simulink model "singleinvertedpendulumsim"  (R2018a)
settings: Solver=FixedStepDiscrete  StartTime=0.0  StopTime=Tsim  FixedStep=Ts  RelTol=1e-3
values from neighbouring files (symbols this model uses):
  K2 = -K2    [singleinvertedpendulum.m]
  R = 0.021    [singleinvertedpendulum.m]
  Ts = 0.001    [singleinvertedpendulum.m]
  x0 = [0;0.1;0;0]    [singleinvertedpendulum.m]
undefined symbols (not defined in the file or in its folder): Ad, Bd, Cd, Dd, Discrete, Ed, Fd, Gd, Hd, Time
libraries: ctrlSharedLib x1, simulink x1
settings Model: Creator=srivats  LastModifiedBy=srivats

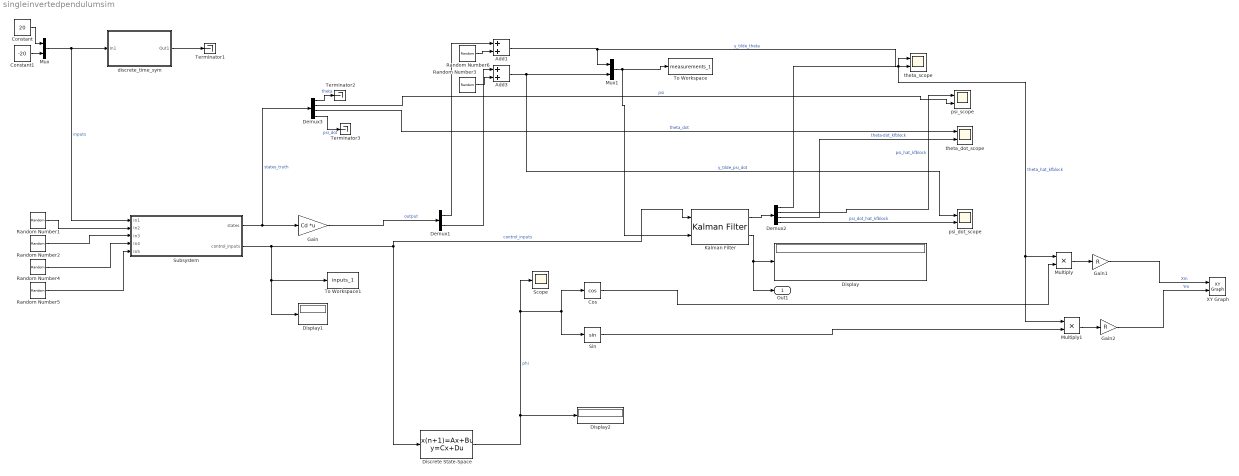
== system singleinvertedpendulumsim ==
  Add1 : Sum
  Add3 : Sum
  Constant : Constant  Value=20
  Constant1 : Constant  Value=-20
  Cos : Trigonometry  Operator=cos
  Demux1 : Demux  Outputs=2
  Demux2 : Demux
  Demux3 : Demux
  Discrete State-Space : DiscreteStateSpace  A=Ed  B=Fd  C=Gd  D=Hd  SampleTime=Ts
  Display : Display
  Display1 : Display
  Display2 : Display
  Gain : Gain  Gain=Cd  Multiplication=Matrix(K*u)
  Gain1 : Gain  Gain=R
  Gain2 : Gain  Gain=R
  Kalman Filter : ctrlSharedLib/Kalman Filter  TimeDomain=Discrete-Time  UseCurrentEstimator=on  ModelSource=Individual A, B, C, D matrices  ModelSourceVariable=ss(0.95,1,1,0,1)  A=Ad  B=Bd  C=Cd  D=Dd  NumberOfStates=4  NumberOfInputs=2  NumberOfOutputs=2  InitialEstimateSource=Dialog  X0=x0  P0=P0  UseK=off  UseGH=off  NumberOfProcessNoiseInputs=1  G=1  TimeInvariantG=on  H=0  TimeInvariantH=on  Q=Q  TimeInvariantQ=on  R=R  TimeInvariantR=on  N=0  TimeInvariantN=on  AddInputPort=on  AddEnablePort=off  OutputEstimatedY=off  OutputP=on  Ts=-1
      settings: SourceProductBaseCode=CT
  Multiply : Product
  Multiply1 : Product
  Mux : Mux  Inputs=2
  Mux1 : Mux  Inputs=2
  Random Number1 : RandomNumber  Variance=0.01  SampleTime=Ts
  Random Number2 : RandomNumber  Variance=0.025  Seed=1  SampleTime=Ts
  Random Number3 : RandomNumber  Variance=0.025  Seed=2  SampleTime=Ts
  Random Number4 : RandomNumber  Variance=0.025  Seed=1  SampleTime=Ts
  Random Number5 : RandomNumber  Variance=0.025  Seed=1  SampleTime=Ts
  Random Number6 : RandomNumber  Variance=0.025  Seed=2  SampleTime=Ts
  Scope : Scope
  Sin : Trigonometry
  Subsystem : Subsystem
  Terminator1 : Terminator
  Terminator2 : Terminator
  Terminator3 : Terminator
  To Workspace : ToWorkspace  VariableName=measurements_1  SaveFormat=Timeseries  SampleTime=-1
  To Workspace1 : ToWorkspace  VariableName=inputs_1  SaveFormat=Timeseries  SampleTime=-1
  XY Graph : simulink/Sinks/XY Graph  xmin=-10  xmax=10  ymin=-10  ymax=10  st=Ts
  discrete_time_sym : Subsystem
  psi_dot_scope : Scope  NumInputPorts=2
  psi_scope : Scope  NumInputPorts=2
  theta_dot_scope : Scope  NumInputPorts=2
  theta_scope : Scope  NumInputPorts=2
  Out1 : Outport
  wires:
  Mux/1 -> Subsystem/1(In1), discrete_time_sym/1(In1)  "inputs"
  Random Number2/1 -> Subsystem/3(In3)
  Random Number1/1 -> Subsystem/2(In2)
  Add3/1 -> psi_dot_scope/1, Mux1/2  "y_tilde_psi_dot"
  Random Number3/1 -> Add3/2
  Constant/1 -> Mux/1
  Constant1/1 -> Mux/2
  Random Number4/1 -> Subsystem/4(In4)
  Random Number5/1 -> Subsystem/5(In5)
  Subsystem/1(states) -> Demux3/1, Gain/1  "states_truth"
  Gain/1 -> Demux1/1  "output"
  Kalman Filter/1 -> Demux2/1
  Demux1/1 -> Add1/1
  Demux1/2 -> Add3/1
  Random Number6/1 -> Add1/2
  Add1/1 -> theta_scope/2, Mux1/1  "y_tilde_theta"
  Subsystem/2(control_inputs) -> Display1/1, To Workspace1/1, Discrete State-Space/1, Kalman Filter/1  "control_inputs"
  Demux2/4 -> psi_dot_scope/2  "psi_dot_hat_kfblock"
  Demux2/3 -> theta_dot_scope/2  "theta-dot_kfblock"
  Demux2/2 -> psi_scope/1  "psi_hat_kfblock"
  Demux2/1 -> theta_scope/1, Multiply1/1, Multiply/1  "theta_hat_kfblock"
  Demux3/2 -> psi_scope/2  "psi"
  Demux3/3 -> theta_dot_scope/1  "theta_dot"
  Demux3/1 -> Terminator2/1  "theta"
  Demux3/4 -> Terminator3/1  "psi_dot"
  discrete_time_sym/1(Out1) -> Terminator1/1
  Kalman Filter/2 -> Out1/1, Display/1
  Mux1/1 -> Kalman Filter/2, To Workspace/1
  Discrete State-Space/1 -> Display2/1, Scope/1, Sin/1, Cos/1  "phi"
  Cos/1 -> Multiply/2
  Multiply/1 -> Gain1/1
  Gain1/1 -> XY Graph/1  "Xm"
  Multiply1/1 -> Gain2/1
  Sin/1 -> Multiply1/2
  Gain2/1 -> XY Graph/2  "Ym"

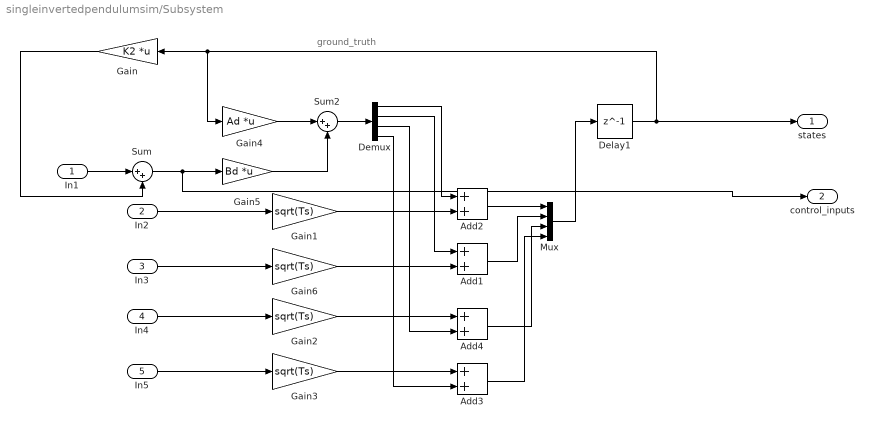
== system singleinvertedpendulumsim/Subsystem ==
  note: ground_truth
  In1 : Inport
  In2 : Inport  Port=2
  In3 : Inport  Port=3
  In4 : Inport  Port=4
  In5 : Inport  Port=5
  Add{1..4} (4 alike) : Sum
  Delay1 : Delay  DelayLength=1  InitialCondition=x0  SampleTime=Ts
  Demux : Demux
  Gain : Gain  Gain=K2  Multiplication=Matrix(K*u)
  Gain{1..3,6} (4 alike) : Gain  Gain=sqrt(Ts)
  Gain4 : Gain  Gain=Ad  Multiplication=Matrix(K*u)
  Gain5 : Gain  Gain=Bd  Multiplication=Matrix(K*u)
  Mux : Mux
  Sum : Sum  Inputs=|++
  Sum2 : Sum  Inputs=|++
  states : Outport
  control_inputs : Outport  Port=2
  wires:
  Add1/1 -> Mux/2
  Gain4/1 -> Sum2/1
  Demux/2 -> Add1/1
  Gain1/1 -> Add2/2
  Sum2/1 -> Demux/1
  Add2/1 -> Mux/1
  Gain6/1 -> Add1/2
  In3/1 -> Gain6/1
  Mux/1 -> Delay1/1
  In2/1 -> Gain1/1
  Gain5/1 -> Sum2/2
  Demux/1 -> Add2/1
  In5/1 -> Gain3/1
  In4/1 -> Gain2/1
  Gain3/1 -> Add3/1
  Gain2/1 -> Add4/1
  Demux/3 -> Add4/2
  Demux/4 -> Add3/2
  Add4/1 -> Mux/3
  Add3/1 -> Mux/4
  In1/1 -> Sum/1
  Delay1/1 -> states/1, Gain/1, Gain4/1
  Gain/1 -> Sum/2
  Sum/1 -> control_inputs/1, Gain5/1

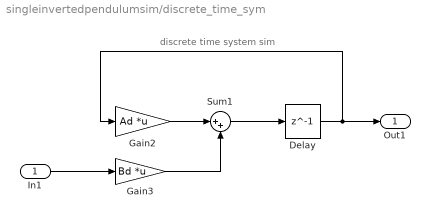
== system singleinvertedpendulumsim/discrete_time_sym ==
  note: discrete time system sim
  In1 : Inport
  Delay : Delay  DelayLength=1  InitialCondition=x0  SampleTime=Ts
  Gain2 : Gain  Gain=Ad  Multiplication=Matrix(K*u)
  Gain3 : Gain  Gain=Bd  Multiplication=Matrix(K*u)
  Sum1 : Sum  Inputs=|++
  Out1 : Outport
  wires:
  Gain3/1 -> Sum1/2
  Sum1/1 -> Delay/1
  Gain2/1 -> Sum1/1
  Delay/1 -> Out1/1, Gain2/1
  In1/1 -> Gain3/1
